simulink model "TEST"  (Simulink 7.7)
settings: Solver=ode45  StartTime=0.0  StopTime=10  RelTol=1e-3
undefined symbols (not defined in the file or in its folder): quad
libraries: simulink x4, fuzblock x1
settings Model: Creator=Alexey  LastModifiedBy=Alexey

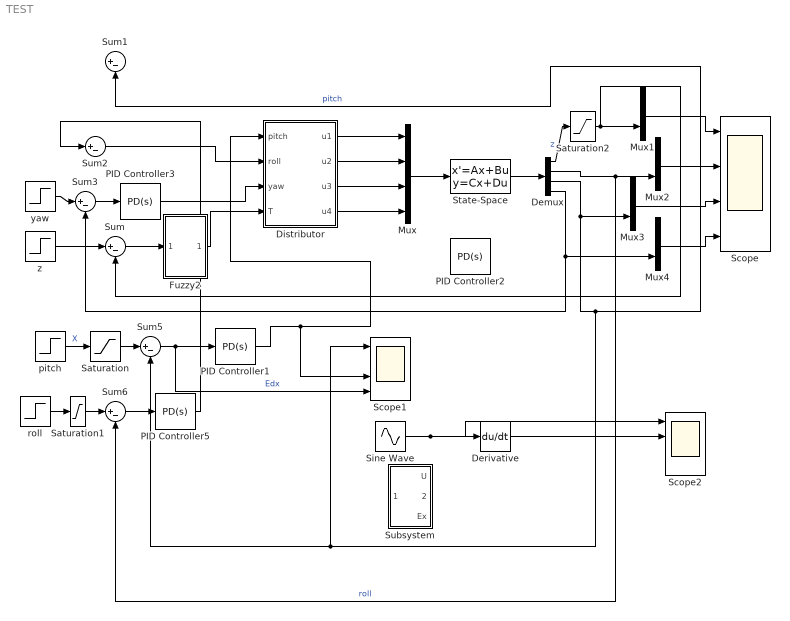
== system TEST ==
  Demux : Demux
  Derivative : Derivative
  Distributor : Subsystem
  Fuzzy2 : Subsystem
  Mux : Mux
  Mux{1..4} (4 alike) : Mux  Inputs=2
  PID Controller1 : simulink/Continuous/PID Controller  SystemSampleTime=-1  Controller=PD  TimeDomain=Continuous-time  SampleTime=1  IntegratorMethod=Forward Euler  FilterMethod=Forward Euler  Form=Parallel  P=0.1  I=0  D=0.4  N=100  InitialConditionSource=internal  InitialConditionForIntegrator=0  InitialConditionForFilter=0  ExternalReset=none  LimitOutput=off  UpperSaturationLimit=inf  LowerSaturationLimit=-inf  LinearizeAsGain=off  AntiWindupMode=none  Kb=1  TrackingMode=off  Kt=1  PParamMin=[]  PParamMax=[]  IParamMin=[]  IParamMax=[]  DParamMin=[]  DParamMax=[]  NParamMin=[]  NParamMax=[]  KbParamMin=[]  KbParamMax=[]  KtParamMin=[]  KtParamMax=[]  POutMin=[]  POutMax=[]  IOutMin=[]  IOutMax=[]  DOutMin=[]  DOutMax=[]  NOutMin=[]  NOutMax=[]  KbOutMin=[]  KbOutMax=[]  KtOutMin=[]  KtOutMax=[]  IntegratorOutMin=[]  IntegratorOutMax=[]  FilterOutMin=[]  FilterOutMax=[]  SumOutMin=[]  SumOutMax=[]  SumI1OutMin=[]  SumI1OutMax=[]  SumI2OutMin=[]  SumI2OutMax=[]  SumI3OutMin=[]  SumI3OutMax=[]  SumDOutMin=[]  SumDOutMax=[]  SaturationOutMin=[]  SaturationOutMax=[]  IntegratorContinuousStateAttributes=''  IntegratorStateMustResolveToSignalObject=off  IntegratorRTWStateStorageClass=Auto  FilterContinuousStateAttributes=''  FilterStateMustResolveToSignalObject=off  FilterRTWStateStorageClass=Auto
  PID Controller2 : simulink/Continuous/PID Controller  SystemSampleTime=-1  Controller=PD  TimeDomain=Continuous-time  SampleTime=1  IntegratorMethod=Forward Euler  FilterMethod=Forward Euler  Form=Parallel  P=50  I=0  D=10  N=100  InitialConditionSource=internal  InitialConditionForIntegrator=0  InitialConditionForFilter=0  ExternalReset=none  LimitOutput=off  UpperSaturationLimit=inf  LowerSaturationLimit=-inf  LinearizeAsGain=off  AntiWindupMode=none  Kb=1  TrackingMode=off  Kt=1  PParamMin=[]  PParamMax=[]  IParamMin=[]  IParamMax=[]  DParamMin=[]  DParamMax=[]  NParamMin=[]  NParamMax=[]  KbParamMin=[]  KbParamMax=[]  KtParamMin=[]  KtParamMax=[]  POutMin=[]  POutMax=[]  IOutMin=[]  IOutMax=[]  DOutMin=[]  DOutMax=[]  NOutMin=[]  NOutMax=[]  KbOutMin=[]  KbOutMax=[]  KtOutMin=[]  KtOutMax=[]  IntegratorOutMin=[]  IntegratorOutMax=[]  FilterOutMin=[]  FilterOutMax=[]  SumOutMin=[]  SumOutMax=[]  SumI1OutMin=[]  SumI1OutMax=[]  SumI2OutMin=[]  SumI2OutMax=[]  SumI3OutMin=[]  SumI3OutMax=[]  SumDOutMin=[]  SumDOutMax=[]  SaturationOutMin=[]  SaturationOutMax=[]  IntegratorContinuousStateAttributes=''  IntegratorStateMustResolveToSignalObject=off  IntegratorRTWStateStorageClass=Auto  FilterContinuousStateAttributes=''  FilterStateMustResolveToSignalObject=off  FilterRTWStateStorageClass=Auto
  PID Controller3 : simulink/Continuous/PID Controller  SystemSampleTime=-1  Controller=PD  TimeDomain=Continuous-time  SampleTime=1  IntegratorMethod=Forward Euler  FilterMethod=Forward Euler  Form=Parallel  P=1  I=0  D=4  N=100  InitialConditionSource=internal  InitialConditionForIntegrator=0  InitialConditionForFilter=0  ExternalReset=none  LimitOutput=off  UpperSaturationLimit=inf  LowerSaturationLimit=-inf  LinearizeAsGain=off  AntiWindupMode=none  Kb=1  TrackingMode=off  Kt=1  PParamMin=[]  PParamMax=[]  IParamMin=[]  IParamMax=[]  DParamMin=[]  DParamMax=[]  NParamMin=[]  NParamMax=[]  KbParamMin=[]  KbParamMax=[]  KtParamMin=[]  KtParamMax=[]  POutMin=[]  POutMax=[]  IOutMin=[]  IOutMax=[]  DOutMin=[]  DOutMax=[]  NOutMin=[]  NOutMax=[]  KbOutMin=[]  KbOutMax=[]  KtOutMin=[]  KtOutMax=[]  IntegratorOutMin=[]  IntegratorOutMax=[]  FilterOutMin=[]  FilterOutMax=[]  SumOutMin=[]  SumOutMax=[]  SumI1OutMin=[]  SumI1OutMax=[]  SumI2OutMin=[]  SumI2OutMax=[]  SumI3OutMin=[]  SumI3OutMax=[]  SumDOutMin=[]  SumDOutMax=[]  SaturationOutMin=[]  SaturationOutMax=[]  IntegratorContinuousStateAttributes=''  IntegratorStateMustResolveToSignalObject=off  IntegratorRTWStateStorageClass=Auto  FilterContinuousStateAttributes=''  FilterStateMustResolveToSignalObject=off  FilterRTWStateStorageClass=Auto
  PID Controller5 : simulink/Continuous/PID Controller  SystemSampleTime=-1  Controller=PD  TimeDomain=Continuous-time  SampleTime=1  IntegratorMethod=Forward Euler  FilterMethod=Forward Euler  Form=Parallel  P=0.1  I=0  D=0.5  N=100  InitialConditionSource=internal  InitialConditionForIntegrator=0  InitialConditionForFilter=0  ExternalReset=none  LimitOutput=off  UpperSaturationLimit=inf  LowerSaturationLimit=-inf  LinearizeAsGain=off  AntiWindupMode=none  Kb=1  TrackingMode=off  Kt=1  PParamMin=[]  PParamMax=[]  IParamMin=[]  IParamMax=[]  DParamMin=[]  DParamMax=[]  NParamMin=[]  NParamMax=[]  KbParamMin=[]  KbParamMax=[]  KtParamMin=[]  KtParamMax=[]  POutMin=[]  POutMax=[]  IOutMin=[]  IOutMax=[]  DOutMin=[]  DOutMax=[]  NOutMin=[]  NOutMax=[]  KbOutMin=[]  KbOutMax=[]  KtOutMin=[]  KtOutMax=[]  IntegratorOutMin=[]  IntegratorOutMax=[]  FilterOutMin=[]  FilterOutMax=[]  SumOutMin=[]  SumOutMax=[]  SumI1OutMin=[]  SumI1OutMax=[]  SumI2OutMin=[]  SumI2OutMax=[]  SumI3OutMin=[]  SumI3OutMax=[]  SumDOutMin=[]  SumDOutMax=[]  SaturationOutMin=[]  SaturationOutMax=[]  IntegratorContinuousStateAttributes=''  IntegratorStateMustResolveToSignalObject=off  IntegratorRTWStateStorageClass=Auto  FilterContinuousStateAttributes=''  FilterStateMustResolveToSignalObject=off  FilterRTWStateStorageClass=Auto
  Saturation : Saturate  UpperLimit=1  LowerLimit=-1
  Saturation1 : Saturate  UpperLimit=1  LowerLimit=-1
  Saturation2 : Saturate  UpperLimit=100  LowerLimit=0
  Scope : Scope  NumInputPorts=4
      settings: TimeRange=2  YMin=-3~-1~-1~-5e-019  YMax=0~1~5.55112e-017~2.5e-018
  Scope1 : Scope  NumInputPorts=4
      settings: TimeRange=2  YMin=-500~0~-1~-225  YMax=100~800~1~-75
  Scope2 : Scope  NumInputPorts=4
      settings: TimeRange=2  YMin=-500~0~-1~-225  YMax=100~800~1~-75  SaveName=ScopeData2
  Sine Wave : Sin  SampleTime=0
  State-Space : StateSpace  A=|  B=|  C=|  D=|
      A=|
      | [0     0     0     0     0     0     0     0;
      |      0     0     0     0     0     0     0     0;
      |      0     0     0     0     0     0     0     0;
      |      0     0     0     0     0     0     0     0;
      |      1     0     0     0     0     0     0     0;
      |      0     1     0     0     0     0     0     0;
      |      0     0     1     0     0     0     0     0;
      |      0     0     0     1     0     0     0     0
      | ]
      B=|
      | [1/quad.m*quad.b     0     0     0;
      |      0     0     1/quad.Ixx*quad.b*quad.l     0;
      |      0     0     0     1/quad.Iyy*quad.b*quad.l;
      |      0     1/quad.Izz*quad.k*quad.r     0     0;
      |      0     0     0     0;
      |      0     0     0     0;
      |      0     0     0     0;
      |      0     0     0     0
      | ]
      C=|
      | [0     0     0     0     1     0     0     0;
      |      0     0     0     0     0     1     0     0;
      |      0     0     0     0     0     0     1     0;
      |      0     0     0     0     0     0     0     1
      | ]
      D=|
      | [[0     0     0     0;
      |      0     0     0     0;
      |      0     0     0     0;
      |      0     0     0     0]]
  Subsystem : Subsystem
  Sum{,1..3,5..6} (6 alike) : Sum  Inputs=|+-
  pitch : Step  Time=0  After=0  SampleTime=0
  roll : Step  Time=3  After=0  SampleTime=0
  yaw : Step  Time=2  After=0  SampleTime=0
  z : Step  Time=0  SampleTime=0
  wires:
  State-Space/1 -> Demux/1
  Demux/1 -> Saturation2/1  "z"
  Demux/2 -> Mux2/2, Sum6/2  "roll"
  Demux/3 -> Mux3/2, Sum1/2, Sum5/2, Scope1/1  "pitch"
  Demux/4 -> Sum3/2, Mux4/2
  Mux/1 -> State-Space/1
  Sum/1 -> Fuzzy2/1(In1)
  z/1 -> Sum/1
  Fuzzy2/1(Out1) -> Distributor/4(T)
  Sum2/1 -> Distributor/2(roll)
  PID Controller3/1 -> Distributor/3(yaw)
  Sum3/1 -> PID Controller3/1
  yaw/1 -> Sum3/1
  PID Controller5/1 -> Sum2/1
  Mux1/1 -> Scope/1
  Mux2/1 -> Scope/2
  Mux3/1 -> Scope/3
  Mux4/1 -> Scope/4
  Distributor/1("u1 ") -> Mux/1
  pitch/1 -> Saturation/1  "X"
  roll/1 -> Saturation1/1
  Sum6/1 -> PID Controller5/1
  Sum5/1 -> Scope1/4, PID Controller1/1  "Edx"
  ? -> Scope1/2  "Ex"
  Distributor/2("u2 ") -> Mux/2
  Distributor/4("u4 ") -> Mux/4
  Distributor/3("u3 ") -> Mux/3
  Saturation/1 -> Sum5/1
  Saturation1/1 -> Sum6/1
  Saturation2/1 -> Sum/2, Mux1/2
  Sine Wave/1 -> Derivative/1, Scope2/1
  Derivative/1 -> Scope2/2
  PID Controller1/1 -> Distributor/1(pitch), Scope1/3

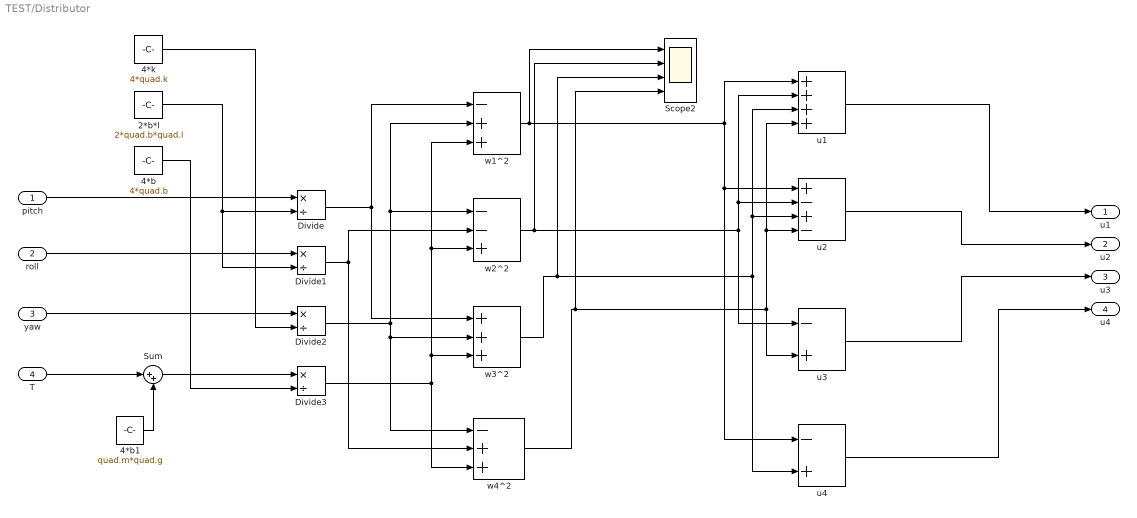
== system TEST/Distributor ==
  pitch : Inport
  roll : Inport  Port=2
  yaw : Inport  Port=3
  T : Inport  Port=4
  2*b*l : Constant  Value=2*quad.b*quad.l
  4*b : Constant  Value=4*quad.b
  4*b1 : Constant  Value=quad.m*quad.g
  4*k : Constant  Value=4*quad.k
  Divide{,1..3} (4 alike) : Product  Inputs=*/
  Scope2 : Scope  NumInputPorts=4
      settings: YMin=-1.5e+007~-2.5e+006~-1.5e+007~-2.5e+006  YMax=2.5e+006~1.25e+007~2.5e+006~1.25e+007  SaveName=ScopeData9
  Sum : Sum  Inputs=|++
  u1 : Sum  Inputs=++++
  u2 : Sum  Inputs=+-+-
  u3 : Sum  Inputs=-+
  u4 : Sum  Inputs=-+
  w1^2 : Sum  Inputs=-++
  w2^2 : Sum  Inputs=--+
  w3^2 : Sum  Inputs=+++
  w4^2 : Sum  Inputs=-++
  "u1 " : Outport
  "u2 " : Outport  Port=2
  "u3 " : Outport  Port=3
  "u4 " : Outport  Port=4
  wires:
  4*k/1 -> Divide2/2
  Divide1/1 -> w4^2/2, w2^2/2
  Divide2/1 -> w3^2/2, w4^2/1, w2^2/1, w1^2/2
  Divide/1 -> w3^2/1, w1^2/1
  4*b/1 -> Divide3/2
  yaw/1 -> Divide2/1
  2*b*l/1 -> Divide/2, Divide1/2
  roll/1 -> Divide1/1
  pitch/1 -> Divide/1
  w1^2/1 -> Scope2/1, u1/1, u2/1, u4/1
  w2^2/1 -> Scope2/2, u1/2, u2/2, u3/1
  w3^2/1 -> Scope2/3, u1/3, u2/3, u4/2
  w4^2/1 -> Scope2/4, u1/4, u2/4, u3/2
  Divide3/1 -> w2^2/3, w1^2/3, w3^2/3, w4^2/3
  u1/1 -> "u1 "/1
  u2/1 -> "u2 "/1
  u3/1 -> "u3 "/1
  u4/1 -> "u4 "/1
  T/1 -> Sum/1
  Sum/1 -> Divide3/1
  4*b1/1 -> Sum/2

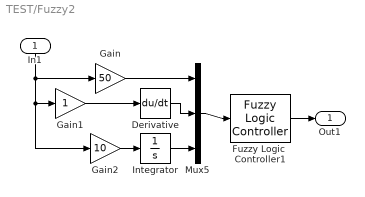
== system TEST/Fuzzy2 ==
  In1 : Inport
  Derivative : Derivative
  Fuzzy Logic  Controller1 : fuzblock/Fuzzy Logic  Controller  SystemSampleTime=-1  fis='Fuzzy.fis'
  Gain : Gain  Gain=50
  Gain1 : Gain
  Gain2 : Gain  Gain=10
  Integrator : Integrator
  Mux5 : Mux  Inputs=3
  Out1 : Outport
  wires:
  Derivative/1 -> Mux5/2
  In1/1 -> Gain1/1, Gain2/1, Gain/1
  Fuzzy Logic  Controller1/1 -> Out1/1
  Integrator/1 -> Mux5/3
  Mux5/1 -> Fuzzy Logic  Controller1/1
  Gain/1 -> Mux5/1
  Gain1/1 -> Derivative/1
  Gain2/1 -> Integrator/1

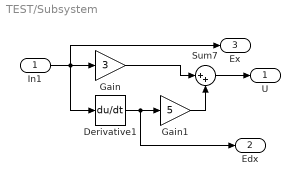
== system TEST/Subsystem ==
  In1 : Inport
  Derivative1 : Derivative
  Gain : Gain  Gain=3
  Gain1 : Gain  Gain=5
  Sum7 : Sum  Inputs=|++
  U : Outport
  Edx : Outport  Port=2
  Ex : Outport  Port=3
  wires:
  In1/1 -> Gain/1, Ex/1, Derivative1/1
  Derivative1/1 -> Gain1/1, Edx/1
  Gain/1 -> Sum7/1
  Sum7/1 -> U/1
  Gain1/1 -> Sum7/2
